simulink model "oMessage_Model"  (R2024b)
settings: Solver=FixedStepDiscrete  StartTime=0.0  StopTime=10.0  FixedStep=0.05  RelTol=1e-3
settings Model: DataDictionary=DataDictionary.sldd  Creator=fl9990  LastModifiedBy=nabilekhoury
settings DataIOCC: SaveOutput=off
settings OptimizationCC: DefaultParameterBehavior=Inlined  OptimizeBlockIOStorage=off  BufferReuse=off  ReuseModelBlockBuffer=off  GlobalBufferReuse=off  ExpressionFolding=off  EnableMemcpy=off  PassReuseOutputArgsAs=Individual arguments  LocalBlockOutputs=off  ZeroExternalMemoryAtStartup=off  ZeroInternalMemoryAtStartup=off  OptimizeDataStoreBuffers=off  BusAssignmentInplaceUpdate=off  OptimizationLevel=level0  OptimizationCustomize=off  EfficientTunableParamExpr=on
settings DebuggingCC: ParameterTunabilityLossMsg=error
settings SFSimCC: MATLABDynamicMemAlloc=off
settings RTWCC: Description=Embedded Coder  SystemTargetFile=ert.tlc  TemplateMakefile=ert_default_tmf  TargetLang=C++
settings CodeAppCC: ForceParamTrailComments=on  IgnoreCustomStorageClasses=off  OperatorAnnotations=on  SimulinkDataObjDesc=on  SFDataObjDesc=on  InsertBlockDesc=on
settings ERTTargetCC: TargetLangStandard=C++17 (ISO)  GenerateSampleERTMain=on  SupportAbsoluteTime=off  CodeInterfacePackaging=C++ class  SupportNonFinite=off  SupportComplex=off  RootIOFormat=Structure reference  ERTCustomFileTemplate=example_file_process.tlc

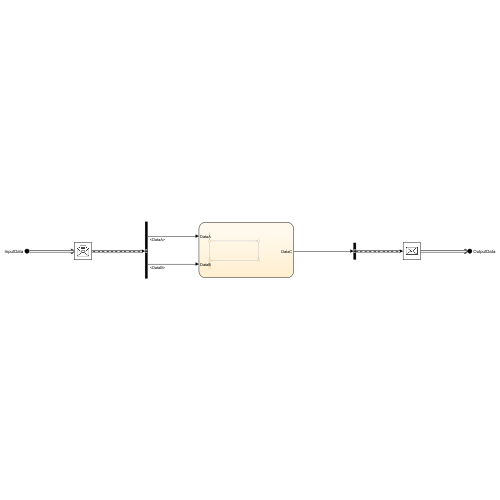
[thumbnail: Simulink's stored preview of the top-level diagram]
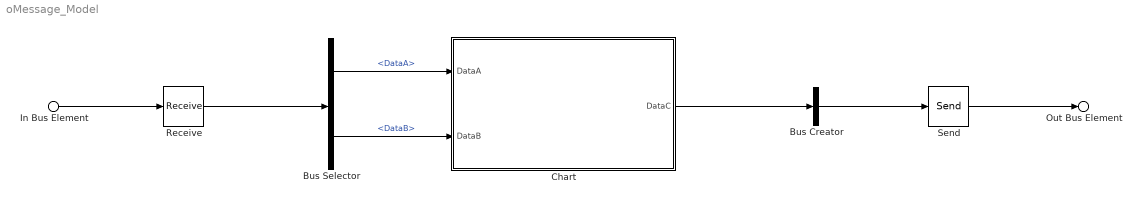
== system oMessage_Model ==
  In Bus Element : Inport  PortName=InputData
  Bus Creator : BusCreator  Inputs=1  OutDataTypeStr=Bus: OutputDataInterface  NonVirtualBus=on
      settings: InheritFromInputs=off
  Bus Selector : BusSelector  OutputSignals=DataA,DataB
  Chart : Stateflow chart  TreatAsAtomicUnit=on
  Receive : Receive  InputPortMessageModes=m  UseInternalQueue=off  QueueOverwriting=on  QueueLength=1  QueueType=LIFO
  Send : Send  OutputPortMessageModes=m
  Out Bus Element : Outport  InputPortMessageModes=m  PortName=OutputData
  wires:
  In Bus Element/1 -> Receive/1
  Chart/1(DataC) -> Bus Creator/1
  Send/1 -> Out Bus Element/1
  Receive/1 -> Bus Selector/1
  Bus Selector/1 -> Chart/1(DataA)  "<DataA>"
  Bus Selector/2 -> Chart/2(DataB)  "<DataB>"
  Bus Creator/1 -> Send/1

== stateflow chart oMessage_Model/Chart ==
  (default) -> (junction 10)
  (junction 10) -> (junction 11) [order 1] : [DataA > 5]
  (junction 10) -> (junction 12) [order 2] : {
      | DataC = DataA * DataB;
      | }
  (junction 11) -> (junction 13) : {
      | DataC = DataA + DataB;
      | }
  (junction 13) -> (junction 12)
  (junction 12) -> (junction 14)
  data: DataA input; DataB input; DataC output
